simulink model "Nealinearni_realni"  (R2023b)
settings: Solver=ode23t  StartTime=0.0  StopTime=10  RelTol=1e-3
values from neighbouring files (symbols this model uses):
  pv_data =     [CNC110X69-5.mat]
undefined symbols (not defined in the file or in its folder): Ci, Cu, D0_ccm, D1, D2, Ipv0, L, pv_eq, RL, step_time, T
libraries: spsSeriesRLCBranchLib x4, spsCurrentMeasurementLib x3, spsVoltageMeasurementLib x2, dspstat3 x2, spsDiodeLib x1, spsControlledCurrentSourceLib x1, spsIdealSwitchLib x1, simulink x1, sps_lib x1
settings Model: Creator=teo  LastModifiedBy=teo

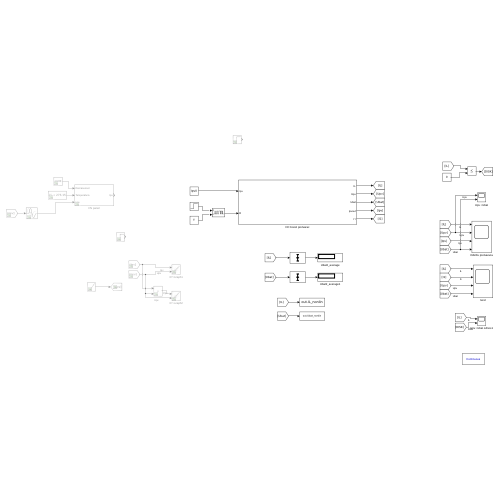
[thumbnail: Simulink's stored preview of the top-level diagram]
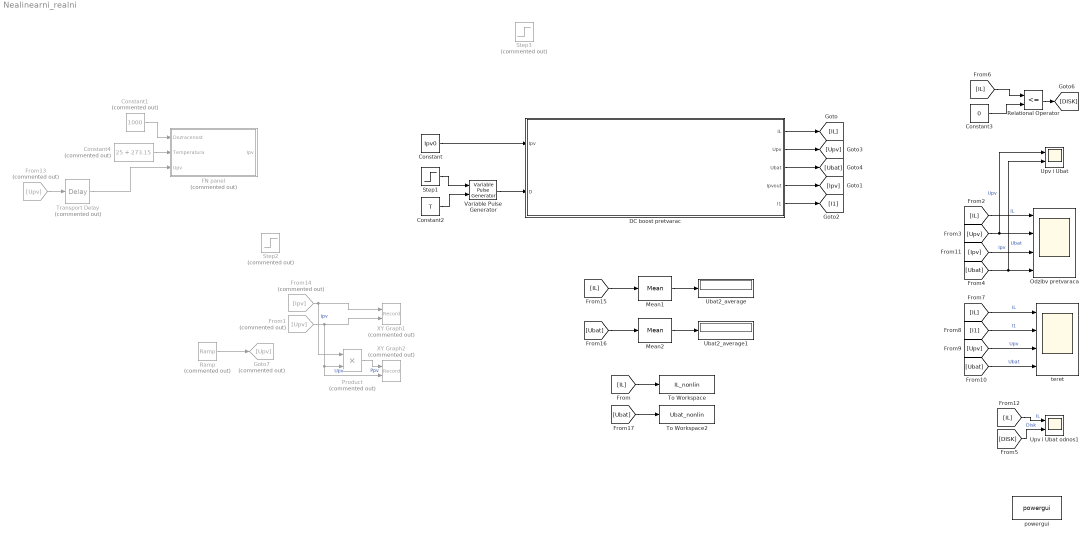
== system Nealinearni_realni ==
  Constant : Constant  Value=Ipv0
  Constant1 : Constant  Commented=on  Value=1000
  Constant2 : Constant  Value=T
  Constant3 : Constant  Value=0
  Constant4 : Constant  Commented=on  Value=25 + 273.15
  DC boost pretvarac : Subsystem
  FN panel : Subsystem  Commented=on
  From1 : From  Commented=on  GotoTag=Upv
  From13 : From  Commented=on  GotoTag=Upv
  From14 : From  Commented=on  GotoTag=Ipv
  Goto7 : Goto  Commented=on  GotoTag=Upv
  Mean1 : dspstat3/Mean  run=off  InputProcessing=Columns as channels (frame based)  reset_popup=None  directionMode=Entire input  dimension=1  roiEnable=off  roiType=Rectangles  roiPortion=Entire ROI  roiOutput=Individual statistics for each ROI  roiFlag=off  roundingMode=Floor  overflowMode=off  outputDataTypeStr=Inherit: Same as accumulator  outputMin=[]  outputMax=[]  outputLastDataTypeStr=Inherit: Same as accumulator
  Mean2 : dspstat3/Mean  run=off  InputProcessing=Columns as channels (frame based)  reset_popup=None  directionMode=Entire input  dimension=1  roiEnable=off  roiType=Rectangles  roiPortion=Entire ROI  roiOutput=Individual statistics for each ROI  roiFlag=off  roundingMode=Floor  overflowMode=off  outputDataTypeStr=Inherit: Same as accumulator  outputMin=[]  outputMax=[]  outputLastDataTypeStr=Inherit: Same as accumulator
  Odzibv pretvaraca : Scope  NumInputPorts=4
  Product : Product  Commented=on
  Ramp : simulink/Sources/Ramp  Commented=on  slope=0.62  start=0  InitialOutput=0
  Relational Operator : RelationalOperator  Operator=<=  OutDataTypeStr=boolean  RndMeth=Simplest  InputSameDT=off
  Step1 : Step  Time=step_time  Before=D1  After=D2  SampleTime=0
  Step2 : Step  Commented=on  Time=5  Before=D0_ccm  After=D0_ccm  SampleTime=0
  Step3 : Step  Commented=on  Time=5  Before=0.4  After=0.75  SampleTime=0
  To Workspace : ToWorkspace  VariableName=IL_nonlin  SaveFormat=Timeseries  SampleTime=-1
  To Workspace2 : ToWorkspace  VariableName=Ubat_nonlin  SaveFormat=Timeseries  SampleTime=-1
  Transport Delay : TransportDelay  Commented=on  DelayTime=0.0001
  Ubat2_average : Display
  Ubat2_average1 : Display
  Upv i Ubat : Scope  NumInputPorts=2
  Upv i Ubat odnos1 : Scope  NumInputPorts=2
  Variable Pulse Generator : VariablePulseGenerator  SampleTime=0.1
  XY Graph1 : Record  Commented=on  FileSettingsInternal="{\"entries\":[{\"content\":{\"excelSettings\":{\"content\":{},\"type\":\"Streamout.ExcelSettings\"}},\"type\":\"Streamout.FileSettingStorage\",\"uuid\":\"\"}],\"packageUris\":[\"http:\\/\\/schema.mathworks.com\\/mf0\\/streamout_blocks\\/R2020a\"],\"version\":\"1.0\"}"  Layout=[1 1]  SignalsInternal="{\"entries\":[{\"content\":{\"signals\":[{\"content\":{\"blockPath\":[],\"dimensions\":[1],\"domain\":\"\",\"lineColor\":\"#edb120\",\"plots\":[1],\"port\":1,\"signalID\":679,\"signalName\":\"Ipv\"},\"type\":\"RecordBlkView.Signal\",\"uuid\":\"\"},{\"content\":{\"blockPath\":[],\"dimensions\":[1],\"domain\":\"\",\"lineColor\":\"#7e2f8e\",\"plots\":[1],\"port\":2,\"signalID\":682,\"signalName\":\"Upv\"},\"type\":\"RecordBlkView.Signal\",\"uuid\":\"\"}]},\"type\":\"RecordBlkView.InputSignals\",\"uuid\":\"\"}],\"packageUris\":[\"http:\\/\\/schema.mathworks.com\\/mf0\\/streamout_blocks\\/R2020a\"],\"version\":\"1.0\"}"  VisualizationBindings="{\"xyplotplugin\":{\"info\":[{\"series\":[{\"bindingParametersList\":[{\"parameter\":\"X-Axis\",\"signalID\":682,\"signalName\":\"Upv\"},{\"parameter\":\"Y-Axis\",\"signalID\":679,\"signalName\":\"Ipv\"}],\"seriesID\":40711}],\"subplotID\":1}]}}"  CompatibilityTag=XY  st=-1
  XY Graph2 : Record  Commented=on  VariableName=PV_record  Filename=Solar_800W.mldatx  FileSettingsInternal="{\"entries\":[{\"content\":{\"excelSettings\":{\"content\":{},\"type\":\"Streamout.ExcelSettings\"}},\"type\":\"Streamout.FileSettingStorage\",\"uuid\":\"\"}],\"packageUris\":[\"http:\\/\\/schema.mathworks.com\\/mf0\\/streamout_blocks\\/R2020a\"],\"version\":\"1.0\"}"  Layout=[1 1]  SignalsInternal="{\"entries\":[{\"content\":{\"signals\":[{\"content\":{\"blockPath\":[],\"dimensions\":[1],\"domain\":\"\",\"lineColor\":\"#77ac30\",\"plots\":[1],\"port\":1,\"signalID\":671,\"signalName\":\"Ppv\"},\"type\":\"RecordBlkView.Signal\",\"uuid\":\"\"},{\"content\":{\"blockPath\":[],\"dimensions\":[1],\"domain\":\"\",\"lineColor\":\"#4dbeee\",\"plots\":[1],\"port\":2,\"signalID\":674,\"signalName\":\"Upv\"},\"type\":\"RecordBlkView.Signal\",\"uuid\":\"\"}]},\"type\":\"RecordBlkView.InputSignals\",\"uuid\":\"\"}],\"packageUris\":[\"http:\\/\\/schema.mathworks.com\\/mf0\\/streamout_blocks\\/R2020a\"],\"version\":\"1.0\"}"  VisualizationBindings="{\"xyplotplugin\":{\"info\":[{\"series\":[{\"bindingParametersList\":[{\"parameter\":\"X-Axis\",\"signalID\":674,\"signalName\":\"Upv\"},{\"parameter\":\"Y-Axis\",\"signalID\":671,\"signalName\":\"Ppv\"}],\"seriesID\":59145}],\"subplotID\":1}]}}"  CompatibilityTag=XY  st=-1
  powergui : sps_lib/powergui  Priority=1  SimulationMode=Continuous  SampleTime=50e-6  frequency=60  Iterations=50  frequencyindice=0  Pbase=100e6  ErrMax=1e-4  UnitsV=kV  UnitsW=MW  buscounter=0  FunctionMessages=off  echomessages=off  EnableUseOfTLC=off  CurrentSourceSwitches=off  DisableSnubberDevices=off  DisableRonSwitches=off  DisableVfSwitches=off  DisplayEquations=off  AutomaticDiscreteSolvers=off  SolverType=Tustin/Backward Euler (TBE)  Interpol=off  ExternalGateDelay=off  methode=off  Ts=100  x0status=blocks  SPID=on  SwTol=0  HookPort=off  NonlinearTolerance=1e-4  nMaxIteration=100  ContinueOnMaxIteration=off  RestoreLinks=warning  ResistiveCurrentMeasurement=off  Frange=[0:2:500]  Ylog=off  Xlog=on  ShowGrid=off  save=off  variable=ZData  structure=0  ZoomFFT=off  StartTime=0.0  cycles=1  DisplayStyle=1  fundamental=60  FreqAxis=off  MaxFrequency=1000  frequencyindicesteady=1  RmsSteady=1  display=off
  teret : Scope  NumInputPorts=4
  wires:
  Constant2/1 -> Variable Pulse Generator/2
  [IL] -> Odzibv pretvaraca/1  "IL"
  [Upv] -> Upv i Ubat/1, Odzibv pretvaraca/2  "Upv"
  [IL] -> teret/1  "IL"
  [I1] -> teret/2  "I1"
  [Upv] -> teret/3  "Upv"
  [IL] -> Upv i Ubat odnos1/1  "IL"
  [DISK] -> Upv i Ubat odnos1/2  "Disk"
  [Ipv] -> Odzibv pretvaraca/3  "Ipv"
  [IL] -> Relational Operator/1
  Relational Operator/1 -> [DISK]
  Constant3/1 -> Relational Operator/2
  Variable Pulse Generator/1 -> DC boost pretvarac/2(D)
  [Ubat] -> Upv i Ubat/2, Odzibv pretvaraca/4  "Ubat"
  [Ubat] -> teret/4  "Ubat"
  DC boost pretvarac/2(Upv) -> [Upv]
  DC boost pretvarac/1(IL) -> [IL]
  DC boost pretvarac/3(Ubat) -> [Ubat]
  DC boost pretvarac/4(Ipvout) -> [Ipv]
  Constant4/1 -> FN panel/2(Temperatura)
  Constant1/1 -> FN panel/1(Dozracenost)
  From13/1 -> Transport Delay/1
  DC boost pretvarac/5(I1) -> [I1]
  Product/1 -> XY Graph2/1  "Ppv"
  From14/1 -> Product/1, XY Graph1/1  "Ipv"
  From1/1 -> XY Graph2/2, Product/2, XY Graph1/2  "Upv"
  Ramp/1 -> Goto7/1
  Transport Delay/1 -> FN panel/3(Upv)
  Step1/1 -> Variable Pulse Generator/1
  Constant/1 -> DC boost pretvarac/1(Ipv)
  [IL] -> Mean1/1
  Mean1/1 -> Ubat2_average/1
  [Ubat] -> Mean2/1
  Mean2/1 -> Ubat2_average1/1
  [IL] -> To Workspace/1
  [Ubat] -> To Workspace2/1

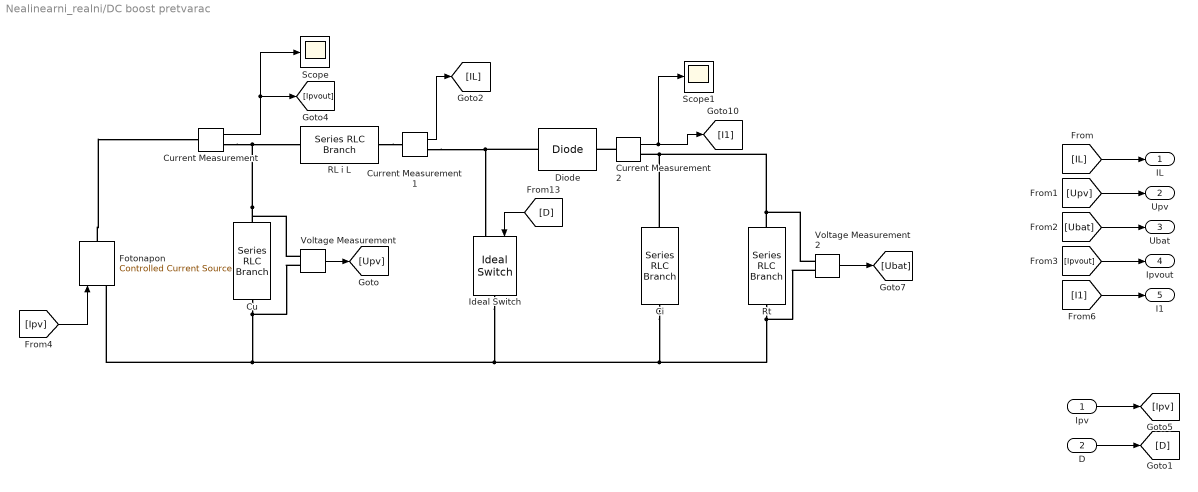
== system Nealinearni_realni/DC boost pretvarac ==
  Ipv : Inport
  D : Inport  Port=2
  Ci : spsSeriesRLCBranchLib/Series RLC Branch  LConnTagsString=__new0  RConnTagsString=__new0  BranchType=RC  Resistance=0.001  Inductance=1e-3  SetiL0=off  InitialCurrent=0  Capacitance=Ci  Setx0=on  InitialVoltage=Ubat0_ccm  Measurements=None
  Cu : spsSeriesRLCBranchLib/Series RLC Branch  LConnTagsString=__new0  RConnTagsString=__new0  BranchType=RC  Resistance=0.001  Inductance=1e-3  SetiL0=off  InitialCurrent=0  Capacitance=Cu  Setx0=on  InitialVoltage=Upv0  Measurements=None
  Current Measurement : spsCurrentMeasurementLib/Current Measurement  PhasorSimulation=off  OutputType=Complex  PSBequivalent=0
  Current Measurement1 : spsCurrentMeasurementLib/Current Measurement  PhasorSimulation=off  OutputType=Complex  PSBequivalent=0
  Current Measurement2 : spsCurrentMeasurementLib/Current Measurement  PhasorSimulation=off  OutputType=Complex  PSBequivalent=0
  Diode : spsDiodeLib/Diode  Ron=0  Lon=0  Vf=0  IC=0  UseSnubber=0  Rs=0  Cs=0  Measurements=off
  Fotonapon : spsControlledCurrentSourceLib/Controlled Current Source  Initialize=on  Source_Type=DC  Amplitude=0  Phase=0  Frequency=0  Measurements=None
  Ideal Switch : spsIdealSwitchLib/Ideal Switch  Ron=0  Lon=0  IC=0  Rs=0  Cs=0  Measurements=off
  RL i L : spsSeriesRLCBranchLib/Series RLC Branch  LConnTagsString=__new0  RConnTagsString=__new0  BranchType=RL  Resistance=RL * 10  Inductance=L  SetiL0=off  InitialCurrent=IL0_ccm  Capacitance=1e-6  Setx0=off  InitialVoltage=0  Measurements=None
  Rt : spsSeriesRLCBranchLib/Series RLC Branch  LConnTagsString=__new0  RConnTagsString=__new0  BranchType=R  Resistance=400  Inductance=1e-3  SetiL0=off  InitialCurrent=0  Capacitance=Ci  Setx0=off  InitialVoltage=0  Measurements=None
  Scope : Scope
  Scope1 : Scope
  Voltage Measurement : spsVoltageMeasurementLib/Voltage Measurement  PhasorSimulation=off  OutputType=Complex  PSBequivalent=0
  Voltage Measurement2 : spsVoltageMeasurementLib/Voltage Measurement  PhasorSimulation=off  OutputType=Complex  PSBequivalent=0
  IL : Outport
  Upv : Outport  Port=2
  Ubat : Outport  Port=3
  Ipvout : Outport  Port=4
  I1 : Outport  Port=5
  wires:
  Current Measurement1/1 -> [IL]
  Voltage Measurement/1 -> [Upv]
  [D] -> Ideal Switch/1
  [Ipv] -> Fotonapon/1
  D/1 -> [D]
  Ipv/1 -> [Ipv]
  [IL] -> IL/1
  [Upv] -> Upv/1
  [Ubat] -> Ubat/1
  Current Measurement/1 -> Scope/1, [Ipvout]
  [Ipvout] -> Ipvout/1
  Current Measurement2/1 -> Scope1/1, [I1]
  Voltage Measurement2/1 -> [Ubat]
  [I1] -> I1/1
  connections:
  Current Measurement/RConn1 -- Voltage Measurement/LConn1 -- Cu/LConn1 -- RL i L/LConn1
  RL i L/RConn1 -- Current Measurement1/LConn1
  Diode/LConn1 -- Ideal Switch/LConn1 -- Current Measurement1/RConn1
  Fotonapon/RConn1 -- Current Measurement/LConn1
  Ideal Switch/RConn1 -- Voltage Measurement2/LConn2 -- Rt/RConn1 -- Ci/RConn1 -- Voltage Measurement/LConn2 -- Cu/RConn1 -- Fotonapon/LConn1
  Ci/LConn1 -- Voltage Measurement2/LConn1 -- Rt/LConn1 -- Current Measurement2/RConn1
  Current Measurement2/LConn1 -- Diode/RConn1

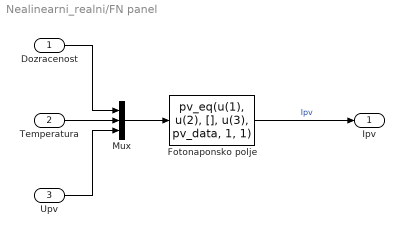
== system Nealinearni_realni/FN panel ==
  Dozracenost : Inport
  Temperatura : Inport  Port=2
  Upv : Inport  Port=3
  Fotonaponsko polje : MATLABFcn  MATLABFcn=pv_eq(u(1), u(2), [], u(3), pv_data, 1, 1)  OutputDimensions=1
  Mux : Mux  Inputs=3
  Ipv : Outport
  wires:
  Fotonaponsko polje/1 -> Ipv/1  "Ipv"
  Mux/1 -> Fotonaponsko polje/1
  Dozracenost/1 -> Mux/1
  Temperatura/1 -> Mux/2
  Upv/1 -> Mux/3
